simulink model "dahlins"  (Simulink 4.00)
settings: Solver=ode45  StartTime=0.0  StopTime=15  FixedStep=0.02  MaxStep=0.02  RelTol=1e-3
settings Model: LastModifiedBy=gordon

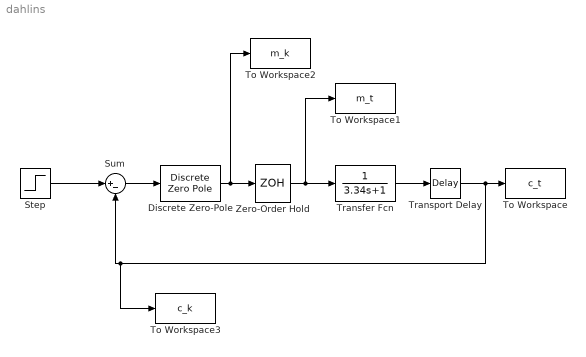
== system dahlins ==
  Discrete Zero-Pole : DiscreteZeroPole  Zeros=[0 0.74]  Poles=[1 -0.39]  Gain=1.526  SampleTime=1
      settings: RTWStateStorageClass=Auto
  Step : Step  Time=2  Before=0  After=1  SampleTime=0
  Sum : Sum  Inputs=|+-  SaturateOnIntegerOverflow=on
  To Workspace : ToWorkspace  VariableName=c_t  SampleTime=0.02  SaveFormat=Array
  To Workspace1 : ToWorkspace  VariableName=m_t  SampleTime=0.02  SaveFormat=Array
  To Workspace2 : ToWorkspace  VariableName=m_k  SampleTime=1  SaveFormat=Array
  To Workspace3 : ToWorkspace  VariableName=c_k  SampleTime=1  SaveFormat=Array
  Transfer Fcn : TransferFcn  Numerator=[1]  Denominator=[3.34 1]  AbsoluteTolerance=auto  Realization=auto
  Transport Delay : TransportDelay  DelayTime=1.46  InitialInput=0  BufferSize=1024  PadeOrder=0
  Zero-Order Hold : ZeroOrderHold  SampleTime=1
  wires:
  Discrete Zero-Pole/1 -> Zero-Order Hold/1, To Workspace2/1
  Sum/1 -> Discrete Zero-Pole/1
  Zero-Order Hold/1 -> Transfer Fcn/1, To Workspace1/1
  Transfer Fcn/1 -> Transport Delay/1
  Transport Delay/1 -> To Workspace/1, Sum/2, To Workspace3/1
  Step/1 -> Sum/1
